simulink model "slip_regulation_stage4"  (R2018a)
settings: Solver=ode4  StartTime=0.0  StopTime=100  FixedStep=0.001  RelTol=1e-3
InitFcn:
  | init_params
values from neighbouring files (symbols this model uses):
  b = 0.1    [init_params.m]
  B0 = 2.5    [init_params.m]
  Is = 0.2    [init_params.m]
  k = 0.4    [init_params.m]
  L = 0.3    [init_params.m]
  m = 100    [init_params.m]
  MFC1 = [9.5 1.9 1.14  0.75]    [init_params.m]
  MFC2 = [2.5 1.8 1 0.2]    [init_params.m]
  MFC3 = [1.5 1.8 0.4 0.2]    [init_params.m]
  N = 500    [init_params.m]
  ppr = 2*pi/1024    (= 0.00613592315154)    [init_params.m]
  R = 3    [init_params.m]
  r = 0.2    [init_params.m]
  Ua = 300    [init_params.m]
  v0 = 1    [init_params.m]
libraries: simulink x2, dspfdesign x2
settings Model: Creator=obrusvit  LastModifiedBy=obrusvit

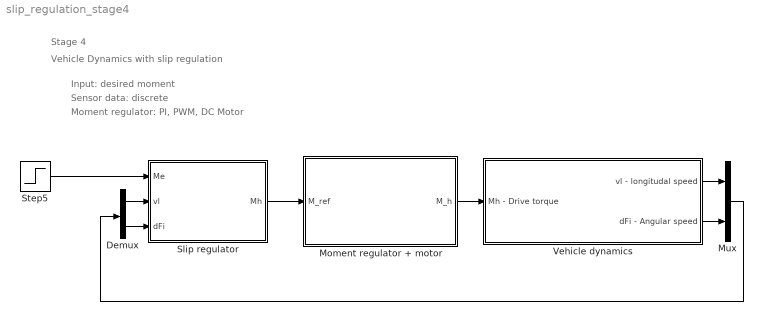
== system slip_regulation_stage4 ==
  note: Stage 4
  note: Moment regulator: PI, PWM, DC Motor
  note: Input: desired moment
  note: Vehicle Dynamics with slip regulation
  note: Sensor data: discrete
  Demux : Demux  Outputs=2
  Moment regulator + motor : Subsystem
  Mux : Mux  Inputs=2
  Slip regulator : Subsystem
  Step5 : Step  Time=0  After=120  SampleTime=0
  Vehicle dynamics : Subsystem
  wires:
  Moment regulator + motor/1("M_h ") -> Vehicle dynamics/1(Mh - Drive torque)
  Vehicle dynamics/2(dFi - Angular speed) -> Mux/2
  Vehicle dynamics/1(vl - longitudal speed) -> Mux/1
  Mux/1 -> Demux/1
  Demux/1 -> Slip regulator/2(vl)
  Demux/2 -> Slip regulator/3(dFi)
  Slip regulator/1("Mh ") -> Moment regulator + motor/1(M_ref)
  Step5/1 -> Slip regulator/1(Me)

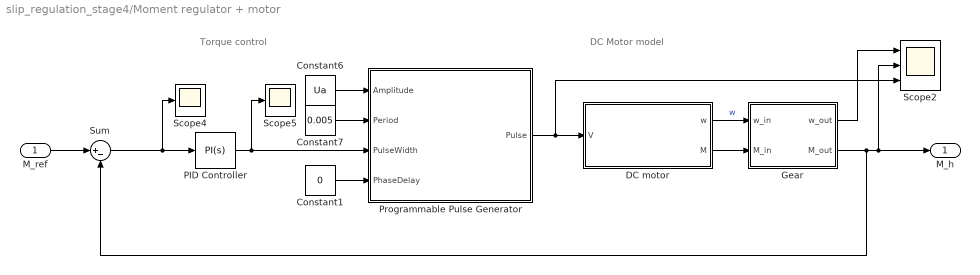
== system slip_regulation_stage4/Moment regulator + motor ==
  note: DC Motor model
  note: Torque control
  M_ref : Inport
  Constant1 : Constant  Value=0
  Constant6 : Constant  Value=Ua
  Constant7 : Constant  Value=0.005
  DC motor : Subsystem  mask(DC Motor){L=L, Kphi=k, J=Is, b=b, R=R}
      mask help:
      | Takes the DC voltage as input, and outputs angular velocity (w) and current (i)
      | L => windings inductance		Kphi => emf constant
      | J => loads moment of inertial		b => viscous friction
      | R => windings resistance
      mask Display:
      | port_label('input', 1, 'V')
      | port_label('output', 1, 'w')
      | port_label('output', 2, 'M')
      | disp('DC Motor')
  Gear : Subsystem
  PID Controller : simulink/Continuous/PID Controller  Controller=PI  TimeDomain=Continuous-time  SampleTime=-1  IntegratorMethod=Forward Euler  FilterMethod=Forward Euler  Form=Parallel  UseFilter=on  ControllerParametersSource=internal  P=5  I=10  D=0  N=100  InitialConditionSource=internal  InitialConditionForIntegrator=0  InitialConditionForFilter=0  ExternalReset=none  ZeroCross=off  LimitOutput=on  UpperSaturationLimit=100  LowerSaturationLimit=0  LinearizeAsGain=on  AntiWindupMode=none  Kb=1  TrackingMode=off  Kt=1  PParamMin=[]  PParamMax=[]  IParamMin=[]  IParamMax=[]  DParamMin=[]  DParamMax=[]  NParamMin=[]  NParamMax=[]  KbParamMin=[]  KbParamMax=[]  KtParamMin=[]  KtParamMax=[]  POutMin=[]  POutMax=[]  IOutMin=[]  IOutMax=[]  DOutMin=[]  DOutMax=[]  NOutMin=[]  NOutMax=[]  KbOutMin=[]  KbOutMax=[]  KtOutMin=[]  KtOutMax=[]  IntegratorOutMin=[]  IntegratorOutMax=[]  FilterOutMin=[]  FilterOutMax=[]  SumOutMin=[]  SumOutMax=[]  SumI1OutMin=[]  SumI1OutMax=[]  SumI2OutMin=[]  SumI2OutMax=[]  SumI3OutMin=[]  SumI3OutMax=[]  SumDOutMin=[]  SumDOutMax=[]  SaturationOutMin=[]  SaturationOutMax=[]  IntegratorContinuousStateAttributes=''  IntegratorStateMustResolveToSignalObject=off  IntegratorRTWStateStorageClass=Auto  FilterContinuousStateAttributes=''  FilterStateMustResolveToSignalObject=off  FilterRTWStateStorageClass=Auto  DifferentiatorICPrevScaledInput=0  DifferentiatorOutMin=[]  DifferentiatorOutMax=[]  FilterDiffOutCoefMin=[]  FilterDiffOutCoefMax=[]  SumDenOutMin=[]  SumDenOutMax=[]  SumNumOutMin=[]  SumNumOutMax=[]  ReciprocalOutMin=[]  ReciprocalOutMax=[]  DivideOutMin=[]  DivideOutMax=[]  TunerSelectOption=Transfer Function Based (PID Tuner App)
  Programmable Pulse Generator : Subsystem
  Scope2 : Scope  NumInputPorts=3
  Scope4 : Scope
  Scope5 : Scope
  Sum : Sum  Inputs=|+-
  "M_h " : Outport
  wires:
  PID Controller/1 -> Programmable Pulse Generator/3(PulseWidth), Scope5/1
  Gear/2(M_out) -> "M_h "/1, Scope2/2, Sum/2
  M_ref/1 -> Sum/1
  Constant7/1 -> Programmable Pulse Generator/2(Period)
  DC motor/2(M) -> Gear/2(M_in)
  Gear/1(w_out) -> Scope2/1
  Sum/1 -> PID Controller/1, Scope4/1
  Programmable Pulse Generator/1(Pulse) -> DC motor/1(V), Scope2/3
  DC motor/1(w) -> Gear/1(w_in)  "w"
  Constant1/1 -> Programmable Pulse Generator/4(PhaseDelay)
  Constant6/1 -> Programmable Pulse Generator/1(Amplitude)

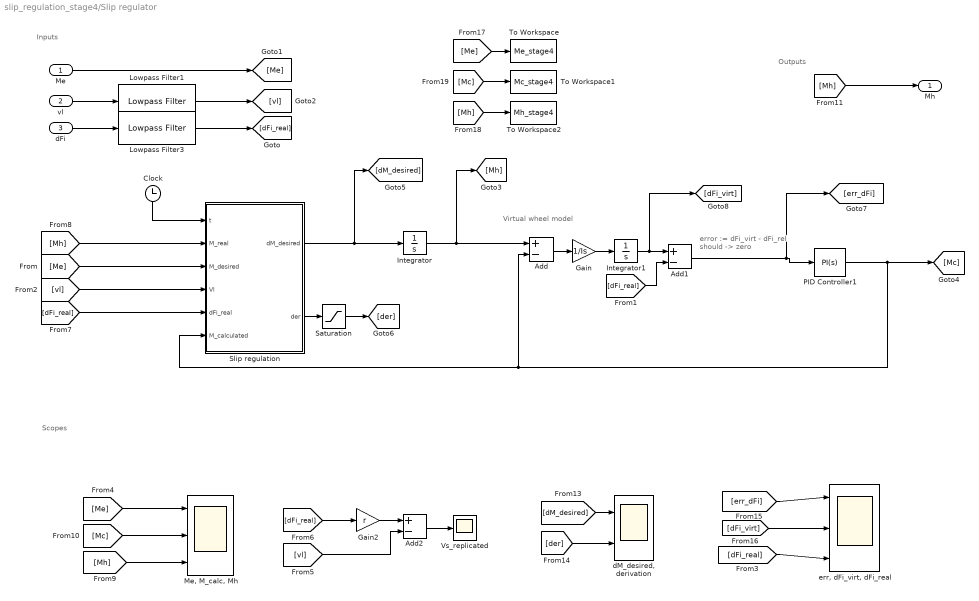
== system slip_regulation_stage4/Slip regulator ==
  note: Scopes
  note: error := dFi_virt - dFi_rel
      | should -> zero
  note: Virtual wheel model
  note: Outputs
  note: Inputs
  Me : Inport
  vl : Inport  Port=2
  dFi : Inport  Port=3
  Add : Sum  Inputs=+-
  Add1 : Sum  Inputs=+-
  Add2 : Sum  Inputs=+-
  Clock : Clock
  Gain : Gain  Gain=1/Is
  Gain2 : Gain  Gain=r
  Integrator : Integrator  LimitOutput=on  LowerSaturationLimit=0
  Integrator1 : Integrator
  Lowpass Filter1 : dspfdesign/Lowpass Filter  FilterType=FIR  DesignForMinimumOrder=off  FilterOrder=50  PassbandFrequency=200  StopbandFrequency=500  PassbandRipple=0.1  StopbandAttenuation=40  InheritSampleRate=off  SampleRate=44100  SimulateUsing=Interpreted execution  roundingMode=Floor  coeffsDataTypeStr=fixdt(1,16)
  Lowpass Filter3 : dspfdesign/Lowpass Filter  FilterType=FIR  DesignForMinimumOrder=off  FilterOrder=50  PassbandFrequency=200  StopbandFrequency=500  PassbandRipple=0.1  StopbandAttenuation=40  InheritSampleRate=off  SampleRate=44100  SimulateUsing=Interpreted execution  roundingMode=Floor  coeffsDataTypeStr=fixdt(1,16)
  "Me, M_calc, Mh" : Scope  NumInputPorts=3
  PID Controller1 : simulink/Continuous/PID Controller  Controller=PI  TimeDomain=Continuous-time  SampleTime=-1  IntegratorMethod=Forward Euler  FilterMethod=Forward Euler  Form=Parallel  UseFilter=on  ControllerParametersSource=internal  P=20  I=20  D=0  N=100  InitialConditionSource=internal  InitialConditionForIntegrator=0  InitialConditionForFilter=0  ExternalReset=none  LimitOutput=on  UpperSaturationLimit=inf  LowerSaturationLimit=0  LinearizeAsGain=on  AntiWindupMode=none  Kb=1  TrackingMode=off  Kt=1  PParamMin=[]  PParamMax=[]  IParamMin=[]  IParamMax=[]  DParamMin=[]  DParamMax=[]  NParamMin=[]  NParamMax=[]  KbParamMin=[]  KbParamMax=[]  KtParamMin=[]  KtParamMax=[]  POutMin=[]  POutMax=[]  IOutMin=[]  IOutMax=[]  DOutMin=[]  DOutMax=[]  NOutMin=[]  NOutMax=[]  KbOutMin=[]  KbOutMax=[]  KtOutMin=[]  KtOutMax=[]  IntegratorOutMin=[]  IntegratorOutMax=[]  FilterOutMin=[]  FilterOutMax=[]  SumOutMin=[]  SumOutMax=[]  SumI1OutMin=[]  SumI1OutMax=[]  SumI2OutMin=[]  SumI2OutMax=[]  SumI3OutMin=[]  SumI3OutMax=[]  SumDOutMin=[]  SumDOutMax=[]  SaturationOutMin=[]  SaturationOutMax=[]  IntegratorContinuousStateAttributes=''  IntegratorStateMustResolveToSignalObject=off  IntegratorRTWStateStorageClass=Auto  FilterContinuousStateAttributes=''  FilterStateMustResolveToSignalObject=off  FilterRTWStateStorageClass=Auto  DifferentiatorICPrevScaledInput=0  DifferentiatorOutMin=[]  DifferentiatorOutMax=[]  FilterDiffOutCoefMin=[]  FilterDiffOutCoefMax=[]  SumDenOutMin=[]  SumDenOutMax=[]  SumNumOutMin=[]  SumNumOutMax=[]  ReciprocalOutMin=[]  ReciprocalOutMax=[]  DivideOutMin=[]  DivideOutMax=[]  TunerSelectOption=Transfer Function Based (PID Tuner App)
  Saturation : Saturate  UpperLimit=1000  LowerLimit=-1000
  Slip regulation : MATLAB Function  TreatAsAtomicUnit=on
  To Workspace : ToWorkspace  VariableName=Me_stage4  SaveFormat=Timeseries  SampleTime=-1
  To Workspace1 : ToWorkspace  VariableName=Mc_stage4  SaveFormat=Timeseries  SampleTime=-1
  To Workspace2 : ToWorkspace  VariableName=Mh_stage4  SaveFormat=Timeseries  SampleTime=-1
  Vs_replicated : Scope
  "dM_desired, derivation " : Scope  NumInputPorts=2
  "err, dFi_virt, dFi_real" : Scope  NumInputPorts=3
  "Mh " : Outport
  wires:
  Me/1 -> [Me]
  [Me] -> Slip regulation/3(M_desired)
  Slip regulation/1(dM_desired) -> [dM_desired], Integrator/1
  Add/1 -> Gain/1
  Gain/1 -> Integrator1/1
  [dFi_real] -> Add1/2
  Integrator1/1 -> [dFi_virt], Add1/1
  [dFi_real] -> "err, dFi_virt, dFi_real"/3
  [Me] -> "Me, M_calc, Mh"/1
  Clock/1 -> Slip regulation/1(t)
  Slip regulation/2(der) -> Saturation/1
  Integrator/1 -> Add/1, [Mh]
  [dFi_real] -> Gain2/1
  [vl] -> Add2/2
  Gain2/1 -> Add2/1
  Add2/1 -> Vs_replicated/1
  PID Controller1/1 -> Add/2, Slip regulation/6(M_calculated), [Mc]
  [vl] -> Slip regulation/4(Vl)
  [dFi_real] -> Slip regulation/5(dFi_real)
  vl/1 -> Lowpass Filter1/1
  Lowpass Filter1/1 -> [vl]
  dFi/1 -> Lowpass Filter3/1
  Lowpass Filter3/1 -> [dFi_real]
  [Mh] -> Slip regulation/2(M_real)
  [Mh] -> "Me, M_calc, Mh"/3
  [Mc] -> "Me, M_calc, Mh"/2
  [Mh] -> "Mh "/1
  [dM_desired] -> "dM_desired, derivation "/1
  Saturation/1 -> [der]
  [der] -> "dM_desired, derivation "/2
  Add1/1 -> [err_dFi], PID Controller1/1
  [err_dFi] -> "err, dFi_virt, dFi_real"/1
  [dFi_virt] -> "err, dFi_virt, dFi_real"/2
  [Me] -> To Workspace/1
  [Mh] -> To Workspace2/1
  [Mc] -> To Workspace1/1

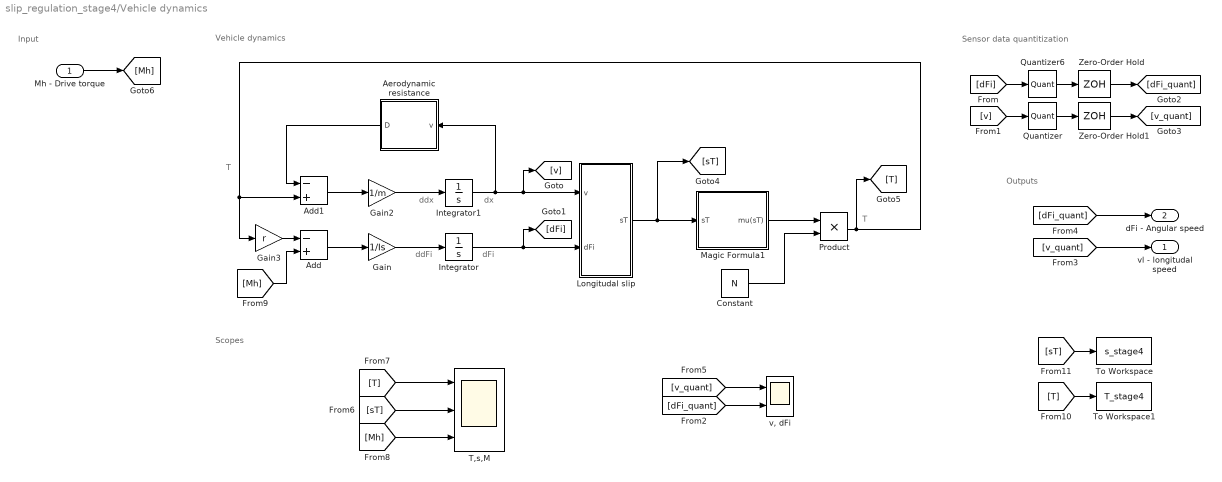
== system slip_regulation_stage4/Vehicle dynamics ==
  note: Sensor data quantitization
  note: Scopes
  note: Outputs
  note: Input
  note: Vehicle dynamics
  note: T
  note: ddx
  note: dx
  note: ddFi
  note: T
  note: dFi
  Mh - Drive torque : Inport
  Add : Sum  Inputs=-+
  Add1 : Sum  Inputs=-+
  "Aerodynamic resistance " : Subsystem
  Constant : Constant  Value=N
  Gain : Gain  Gain=1/Is
  Gain2 : Gain  Gain=1/m
  Gain3 : Gain  Gain=r
  Integrator : Integrator  InitialCondition=v0/r
  Integrator1 : Integrator  InitialCondition=v0
  Longitudal slip : Subsystem
  Magic Formula1 : Subsystem
  Product : Product
  Quantizer : Quantizer  QuantizationInterval=ppr/2
  Quantizer6 : Quantizer  QuantizationInterval=ppr/2
  T,s,M : Scope  NumInputPorts=3
  To Workspace : ToWorkspace  VariableName=s_stage4  SaveFormat=Timeseries  SampleTime=-1
  To Workspace1 : ToWorkspace  VariableName=T_stage4  SaveFormat=Timeseries  SampleTime=-1
  Zero-Order Hold : ZeroOrderHold  SampleTime=0.001
  Zero-Order Hold1 : ZeroOrderHold  SampleTime=0.001
  "v, dFi" : Scope  NumInputPorts=2
  vl - longitudal speed : Outport
  dFi - Angular speed : Outport  Port=2
  wires:
  Longitudal slip/1(sT) -> [sT], Magic Formula1/1(sT)
  Add1/1 -> Gain2/1
  "Aerodynamic resistance "/1("D ") -> Add1/1
  Gain3/1 -> Add/1
  Magic Formula1/1(mu(sT)) -> Product/1
  Gain/1 -> Integrator/1
  Add/1 -> Gain/1
  Constant/1 -> Product/2
  Gain2/1 -> Integrator1/1
  Integrator/1 -> [dFi], Longitudal slip/2(dFi)
  Integrator1/1 -> [v], Longitudal slip/1(v), "Aerodynamic resistance "/1(v)
  Quantizer6/1 -> Zero-Order Hold/1
  Quantizer/1 -> Zero-Order Hold1/1
  Zero-Order Hold1/1 -> [v_quant]
  Zero-Order Hold/1 -> [dFi_quant]
  [dFi] -> Quantizer6/1
  [v] -> Quantizer/1
  [dFi_quant] -> "v, dFi"/2
  [v_quant] -> vl - longitudal speed/1
  [dFi_quant] -> dFi - Angular speed/1
  [v_quant] -> "v, dFi"/1
  [sT] -> T,s,M/2
  Product/1 -> Gain3/1, Add1/2, [T]
  [T] -> T,s,M/1
  Mh - Drive torque/1 -> [Mh]
  [Mh] -> T,s,M/3
  [Mh] -> Add/2
  [sT] -> To Workspace/1
  [T] -> To Workspace1/1

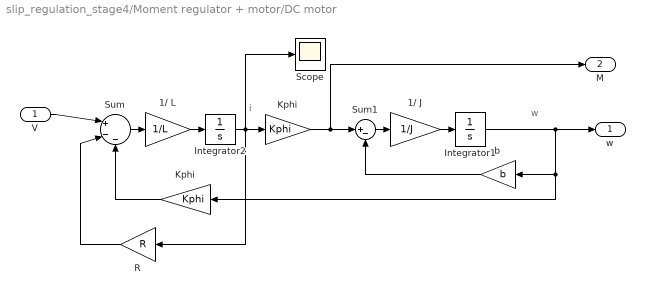
== system slip_regulation_stage4/Moment regulator + motor/DC motor ==
  note: i
  note: w
  V : Inport
  1/ J : Gain  Gain=1/J
  1/ L : Gain  Gain=1/L
  Integrator1 : Integrator
  Integrator2 : Integrator
  Kphi : Gain  Gain=Kphi
  "Kphi " : Gain  Gain=Kphi
  R : Gain  Gain=R
  Scope : Scope
  Sum : Sum  Inputs=|+--
  Sum1 : Sum  Inputs=|+-
  b : Gain  Gain=b
  w : Outport
  M : Outport  Port=2
  wires:
  V/1 -> Sum/1
  Sum/1 -> 1/ L/1
  1/ L/1 -> Integrator2/1
  Integrator2/1 -> Scope/1, Kphi/1, R/1
  Kphi/1 -> M/1, Sum1/1
  Sum1/1 -> 1/ J/1
  1/ J/1 -> Integrator1/1
  b/1 -> Sum1/2
  "Kphi "/1 -> Sum/3
  R/1 -> Sum/2
  Integrator1/1 -> "Kphi "/1, b/1, w/1

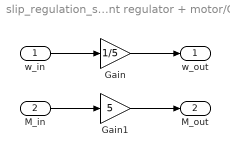
== system slip_regulation_stage4/Moment regulator + motor/Gear ==
  w_in : Inport
  M_in : Inport  Port=2
  Gain : Gain  Gain=1/5
  Gain1 : Gain  Gain=5
  w_out : Outport
  M_out : Outport  Port=2
  wires:
  w_in/1 -> Gain/1
  Gain/1 -> w_out/1
  M_in/1 -> Gain1/1
  Gain1/1 -> M_out/1

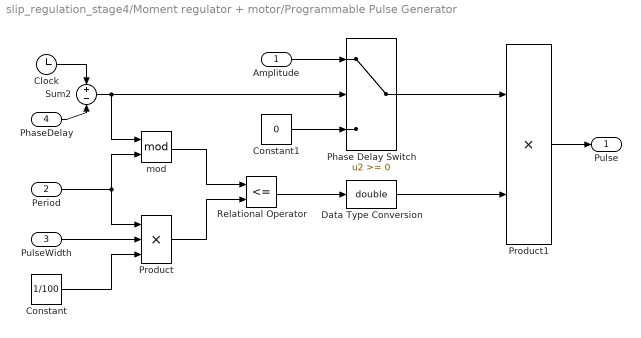
== system slip_regulation_stage4/Moment regulator + motor/Programmable Pulse Generator ==
  Amplitude : Inport
  Period : Inport  Port=2
  PulseWidth : Inport  Port=3
  PhaseDelay : Inport  Port=4
  Clock : Clock
  Constant : Constant  Value=1/100
  Constant1 : Constant  Value=0
  Data Type Conversion : DataTypeConversion  OutDataTypeStr=double
  Phase Delay Switch : Switch
  Product : Product  Inputs=3  RndMeth=Zero
  Product1 : Product  RndMeth=Zero
  Relational Operator : RelationalOperator  Operator=<=  RndMeth=Nearest
  Sum2 : Sum  Inputs=+-
  mod : Math  Operator=mod  SaturateOnIntegerOverflow=on
  Pulse : Outport
  wires:
  Product/1 -> Relational Operator/2
  Product1/1 -> Pulse/1
  Data Type Conversion/1 -> Product1/2
  Relational Operator/1 -> Data Type Conversion/1
  Constant/1 -> Product/3
  PulseWidth/1 -> Product/2
  mod/1 -> Relational Operator/1
  Period/1 -> Product/1, mod/2
  Clock/1 -> Sum2/1
  PhaseDelay/1 -> Sum2/2
  Sum2/1 -> mod/1, Phase Delay Switch/2
  Amplitude/1 -> Phase Delay Switch/1
  Constant1/1 -> Phase Delay Switch/3
  Phase Delay Switch/1 -> Product1/1

== system slip_regulation_stage4/Vehicle dynamics/Aerodynamic resistance  ==
  v : Inport
  Gain1 : Gain  Gain=B0
  Product : Product
  Sign : Signum
  Square : Math  Operator=square  SaturateOnIntegerOverflow=on
  "D " : Outport
  wires:
  v/1 -> Sign/1, Square/1
  Square/1 -> Product/2
  Sign/1 -> Product/1
  Gain1/1 -> "D "/1
  Product/1 -> Gain1/1

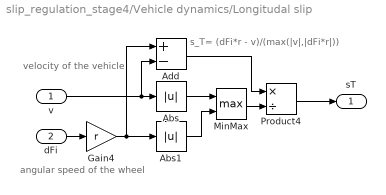
== system slip_regulation_stage4/Vehicle dynamics/Longitudal slip ==
  note: s_T= (dFi*r - v)/(max(|v|,|dFi*r|))
  note: angular speed
      | of the wheel
  note: velocity
      | of the vehicle
  v : Inport
  dFi : Inport  Port=2
  Abs : Abs
  Abs1 : Abs
  Add : Sum  Inputs=+-
  Gain4 : Gain  Gain=r
  MinMax : MinMax  Function=max  Inputs=2
  Product4 : Product  Inputs=*/  RndMeth=Zero
  sT : Outport
  wires:
  Product4/1 -> sT/1
  Add/1 -> Product4/1
  Abs1/1 -> MinMax/2
  Abs/1 -> MinMax/1
  MinMax/1 -> Product4/2
  Gain4/1 -> Add/1, Abs1/1
  dFi/1 -> Gain4/1
  v/1 -> Add/2, Abs/1

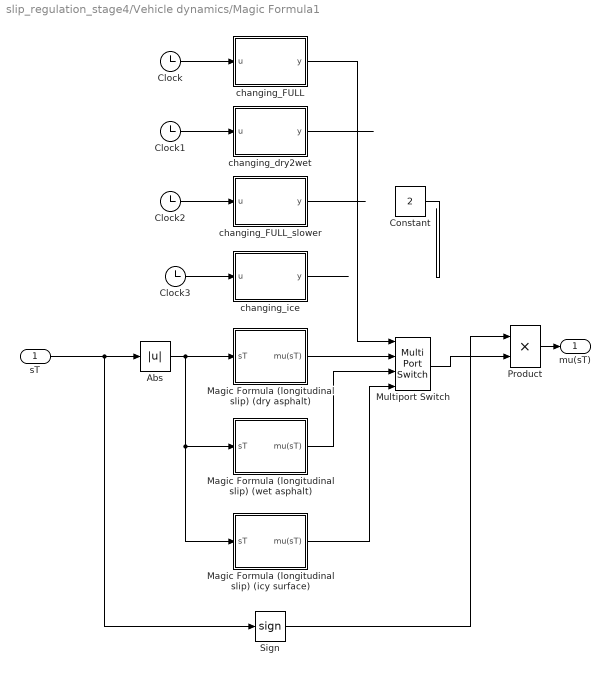
== system slip_regulation_stage4/Vehicle dynamics/Magic Formula1 ==
  sT : Inport
  Abs : Abs
  Clock{,1..3} (4 alike) : Clock
  Constant : Constant  Value=2
  Magic Formula (longitudinal slip) (dry asphalt) : Subsystem
  Magic Formula (longitudinal slip) (icy surface) : Subsystem
  Magic Formula (longitudinal slip) (wet asphalt) : Subsystem
  Multiport Switch : MultiPortSwitch
  Product : Product
  Sign : Signum
  changing_FULL : MATLAB Function  TreatAsAtomicUnit=on
  changing_FULL_slower : MATLAB Function  TreatAsAtomicUnit=on
  changing_dry2wet : MATLAB Function  TreatAsAtomicUnit=on
  changing_ice : MATLAB Function  TreatAsAtomicUnit=on
  mu(sT) : Outport
  wires:
  Abs/1 -> Magic Formula (longitudinal slip) (icy surface)/1(sT), Magic Formula (longitudinal slip) (wet asphalt)/1(sT), Magic Formula (longitudinal slip) (dry asphalt)/1(sT)
  Magic Formula (longitudinal slip) (dry asphalt)/1(mu(sT)) -> Multiport Switch/2
  Product/1 -> mu(sT)/1
  Sign/1 -> Product/1
  sT/1 -> Sign/1, Abs/1
  Magic Formula (longitudinal slip) (wet asphalt)/1(mu(sT)) -> Multiport Switch/3
  Multiport Switch/1 -> Product/2
  Magic Formula (longitudinal slip) (icy surface)/1(mu(sT)) -> Multiport Switch/4
  Clock/1 -> changing_FULL/1(u)
  changing_FULL/1(y) -> Multiport Switch/1
  Constant/1 -> ?
  Clock1/1 -> changing_dry2wet/1(u)
  changing_dry2wet/1(y) -> ?
  Clock2/1 -> changing_FULL_slower/1(u)
  changing_FULL_slower/1(y) -> ?
  Clock3/1 -> changing_ice/1(u)
  changing_ice/1(y) -> ?

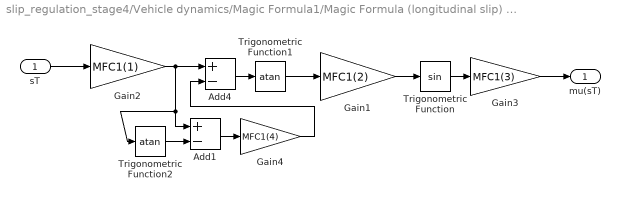
== system slip_regulation_stage4/Vehicle dynamics/Magic Formula1/Magic Formula (longitudinal slip) (dry asphalt) ==
  sT : Inport
  Add1 : Sum  Inputs=+-
  Add4 : Sum  Inputs=+-
  Gain1 : Gain  Gain=MFC1(2)
  Gain2 : Gain  Gain=MFC1(1)
  Gain3 : Gain  Gain=MFC1(3)
  Gain4 : Gain  Gain=MFC1(4)
  Trigonometric Function : Trigonometry
  Trigonometric Function1 : Trigonometry  Operator=atan
  Trigonometric Function2 : Trigonometry  Operator=atan
  mu(sT) : Outport
  wires:
  Gain3/1 -> mu(sT)/1
  sT/1 -> Gain2/1
  Add4/1 -> Trigonometric Function1/1
  Gain4/1 -> Add4/2
  Add1/1 -> Gain4/1
  Trigonometric Function2/1 -> Add1/2
  Gain2/1 -> Trigonometric Function2/1, Add1/1, Add4/1
  Trigonometric Function1/1 -> Gain1/1
  Gain1/1 -> Trigonometric Function/1
  Trigonometric Function/1 -> Gain3/1

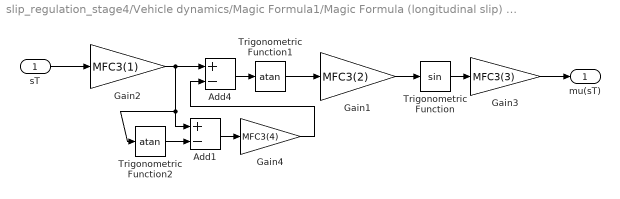
== system slip_regulation_stage4/Vehicle dynamics/Magic Formula1/Magic Formula (longitudinal slip) (icy surface) ==
  sT : Inport
  Add1 : Sum  Inputs=+-
  Add4 : Sum  Inputs=+-
  Gain1 : Gain  Gain=MFC3(2)
  Gain2 : Gain  Gain=MFC3(1)
  Gain3 : Gain  Gain=MFC3(3)
  Gain4 : Gain  Gain=MFC3(4)
  Trigonometric Function : Trigonometry
  Trigonometric Function1 : Trigonometry  Operator=atan
  Trigonometric Function2 : Trigonometry  Operator=atan
  mu(sT) : Outport
  wires:
  Gain3/1 -> mu(sT)/1
  sT/1 -> Gain2/1
  Add4/1 -> Trigonometric Function1/1
  Gain4/1 -> Add4/2
  Add1/1 -> Gain4/1
  Trigonometric Function2/1 -> Add1/2
  Gain2/1 -> Trigonometric Function2/1, Add1/1, Add4/1
  Trigonometric Function1/1 -> Gain1/1
  Gain1/1 -> Trigonometric Function/1
  Trigonometric Function/1 -> Gain3/1

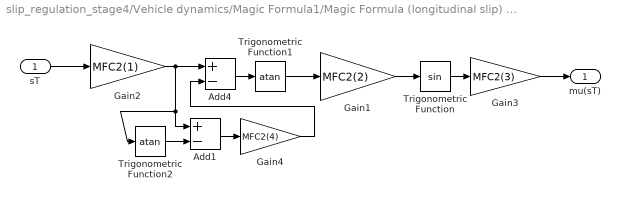
== system slip_regulation_stage4/Vehicle dynamics/Magic Formula1/Magic Formula (longitudinal slip) (wet asphalt) ==
  sT : Inport
  Add1 : Sum  Inputs=+-
  Add4 : Sum  Inputs=+-
  Gain1 : Gain  Gain=MFC2(2)
  Gain2 : Gain  Gain=MFC2(1)
  Gain3 : Gain  Gain=MFC2(3)
  Gain4 : Gain  Gain=MFC2(4)
  Trigonometric Function : Trigonometry
  Trigonometric Function1 : Trigonometry  Operator=atan
  Trigonometric Function2 : Trigonometry  Operator=atan
  mu(sT) : Outport
  wires:
  Gain3/1 -> mu(sT)/1
  sT/1 -> Gain2/1
  Add4/1 -> Trigonometric Function1/1
  Gain4/1 -> Add4/2
  Add1/1 -> Gain4/1
  Trigonometric Function2/1 -> Add1/2
  Gain2/1 -> Trigonometric Function2/1, Add1/1, Add4/1
  Trigonometric Function1/1 -> Gain1/1
  Gain1/1 -> Trigonometric Function/1
  Trigonometric Function/1 -> Gain3/1

== matlab function slip_regulation_stage4/Vehicle dynamics/Magic Formula1/changing_FULL ==
  data: u input; y output
function y = fcn(u)
if u <= 20
    y = 1;
elseif u <= 40
    y = 2;
elseif u <= 60
    y = 3;
elseif u <= 80
    y = 2;
else
    y = 1;
end
end

== matlab function slip_regulation_stage4/Vehicle dynamics/Magic Formula1/changing_dry2wet ==
  data: u input; y output
function y = fcn(u)
if u <= 50
    y = 1;

else
    y = 2;
end
end

== matlab function slip_regulation_stage4/Vehicle dynamics/Magic Formula1/changing_FULL_slower ==
  data: u input; y output
function y = fcn(u)
if u <= 100
    y = 1;
elseif u<=200
    y = 2;
elseif u <= 300
    y = 3;
elseif u <= 400
    y = 2;
else
    y = 1;
end
end

== matlab function slip_regulation_stage4/Slip regulator/Slip regulation ==
  settings: updateMethod=DISCRETE
  data: t input; M_real input; M_desired input; Vl input; dFi_real input; dM_desired output; M_calculated input; der output; par_ctr parameter
function [dM_desired, der] = fcn(t, M_real, M_desired, Vl, dFi_real, M_calculated, par_ctr)

persistent dt;

persistent dT;
persistent dVs;

persistent last_Mcalc;
persistent last_Vs;

persistent last_t;

if isempty(dt)
    dt = 0.01;
end
if isempty(dT)
    dT = M_calculated;
end
if isempty(dVs)
    dVs = 0;
end
if isempty(last_Mcalc)
    last_Mcalc = M_calculated;
end
if isempty(last_Vs)
    last_Vs = 0;
end
if isempty(last_t)
    last_t = t;
end
    
%% Main algorithm

dt = t-last_t;
if dt >= par_ctr.TS

    Vc = dFi_real * par_ctr.r;
    Vs = Vc-Vl; 

    % compute differences and save current values
    dT = M_calculated - last_Mcalc;
    dVs = Vs -last_Vs;
    last_t = t;
    last_Mcalc = M_calculated;
    last_Vs = Vs;


    diff = M_desired - M_calculated;
    der = 0;
    if abs(diff) <= par_ctr.ERR_TOLERABLE       %Force is just OK
        dM_desired = 0;
    elseif diff <= par_ctr.ERR_TOLERABLE        %driver wants to REDUCE force
        dM_desired = -par_ctr.dM_default;
    else                                        %driver wants to INCREASE force  
        if M_calculated == 0
            % get it runnin' booy
            dM_desired = par_ctr.dM_default;
            return
        end
        derivation = dT/dVs;
        der = derivation;
        dM_desired = choose_dM(derivation);

        if (Vs >= par_ctr.CRITICAL_SLIP_VEL)
            % We started to slip too much
            % quickly decrease M_h
            dM_desired = dM_desired - 100;
        end

        if (M_calculated - M_real) >= par_ctr.CRITICAL_M_CALC_REAL_MISMATCH
            % M_real is way below M_calc
            % that means we were slipping
            % but we do not want to drop M to zero
            dM_desired = 0;
        end
    end
else
    dM_desired = 0;
    der = 0;
end


    function dM_chosen = choose_dM(derivation)
        for i = 1:numel(par_ctr.der_TH)
            if derivation >= par_ctr.der_TH(i)
                dM_chosen = par_ctr.dM_val(i);
                return;
            end
        end
        dM_chosen = par_ctr.dM_val(end);
    end

end

== matlab function slip_regulation_stage4/Vehicle dynamics/Magic Formula1/changing_ice ==
  data: u input; y output
function y = fcn(u)
if u <= 50
    y = 1;
else
    y = 3;
end
end
